simulink model "PI"  (R2015a)
settings: Solver=ode45  StartTime=0.0  StopTime=10.0  RelTol=1e-3
libraries: cstblocks x2
settings Model: Creator=Tuor  LastModifiedBy=Tuor

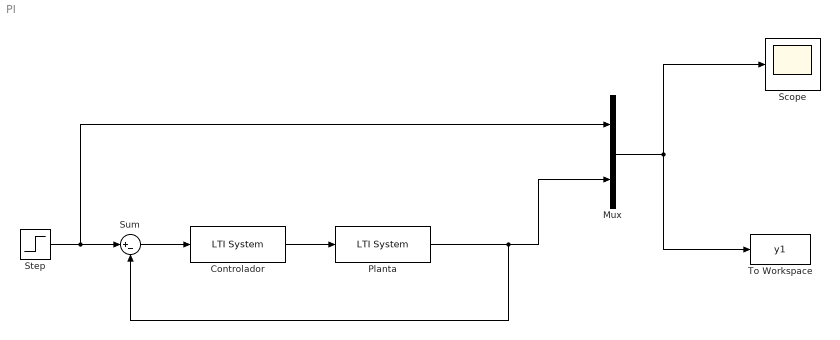
== system PI ==
  Controlador : cstblocks/LTI System  sys=Gc  IC=[]
  Mux : Mux  Inputs=2
  Planta : cstblocks/LTI System  sys=Gp  IC=[]
  Scope : Scope
  Step : Step  SampleTime=0
  Sum : Sum  Inputs=|+-
  To Workspace : ToWorkspace  VariableName=y1  SaveFormat=Timeseries  SampleTime=-1
  wires:
  Step/1 -> Mux/1, Sum/1
  Sum/1 -> Controlador/1
  Controlador/1 -> Planta/1
  Planta/1 -> Sum/2, Mux/2
  Mux/1 -> To Workspace/1, Scope/1
